simulink model "effect_feedback"  (R2023b)
settings: Solver=VariableStepAuto  StartTime=0.0  StopTime=10.0  RelTol=1e-3
settings Model: Creator=hp  LastModifiedBy=hp

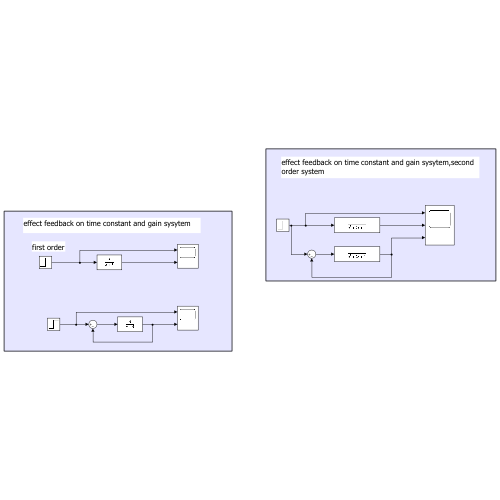
[thumbnail: Simulink's stored preview of the top-level diagram]
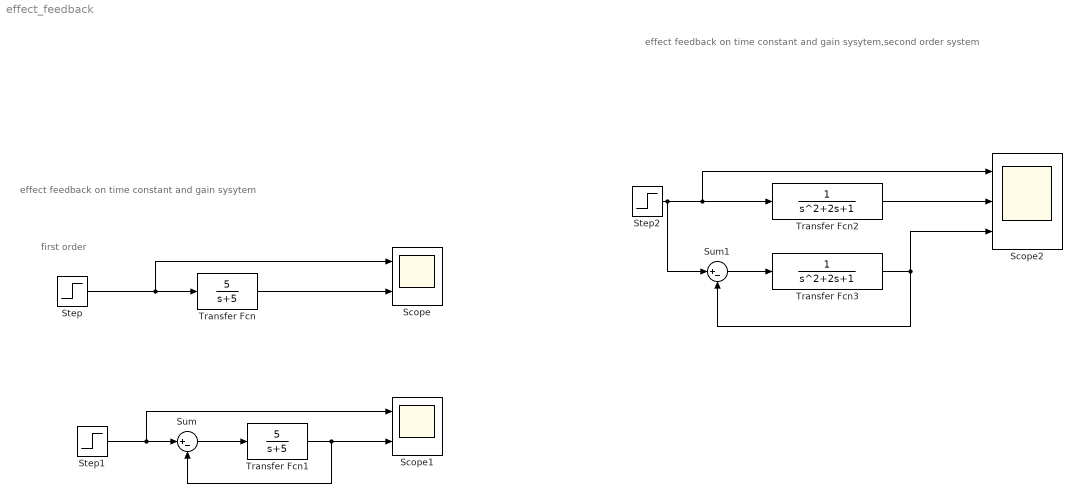
== system effect_feedback ==
  note: effect feedback on time constant and gain sysytem,second order system
  note: first order
  note: effect feedback on time constant and gain sysytem
  Scope : Scope  NumInputPorts=2
  Scope1 : Scope  NumInputPorts=2
  Scope2 : Scope  NumInputPorts=3
  Step : Step  SampleTime=0
  Step1 : Step  SampleTime=0
  Step2 : Step  SampleTime=0
  Sum : Sum  Inputs=|+-
  Sum1 : Sum  Inputs=|+-
  Transfer Fcn : TransferFcn  Numerator=[5]  Denominator=[1 5]
  Transfer Fcn1 : TransferFcn  Numerator=[5]  Denominator=[1 5]
  Transfer Fcn2 : TransferFcn
  Transfer Fcn3 : TransferFcn
  wires:
  Step/1 -> Scope/1, Transfer Fcn/1
  Transfer Fcn/1 -> Scope/2
  Step1/1 -> Scope1/1, Sum/1
  Sum/1 -> Transfer Fcn1/1
  Transfer Fcn1/1 -> Scope1/2, Sum/2
  Transfer Fcn2/1 -> Scope2/2
  Step2/1 -> Sum1/1, Scope2/1, Transfer Fcn2/1
  Sum1/1 -> Transfer Fcn3/1
  Transfer Fcn3/1 -> Scope2/3, Sum1/2
